simulink model "test_model"  (R2019b)
settings: Solver=VariableStepAuto  StartTime=0.0  StopTime=20  RelTol=1e-5
values from neighbouring files (symbols this model uses):
  dq0 = optimization(4:6)    [run_optimization.m]    (also in run_simulation.m = [0; 0; 8]; set_path.m = [0; 0; 8]; test_simulink.m = [0; 0; 8])
  q0 = optimization(1:3)    [run_optimization.m]    (also in run_simulation.m = [pi/9; -pi/9; 0]; set_path.m = [pi/9; -pi/9; 0]; test_simulink.m = [pi/9; -pi/9; 0])
  threshold = 1e-3    (= 0.001)    [test_simulink.m]
  x0 = [q0;dq0]    [set_path.m]    (also in test_simulink.m)
libraries: dspinverses x1
settings Model: Creator=Niilouf  LastModifiedBy=berth

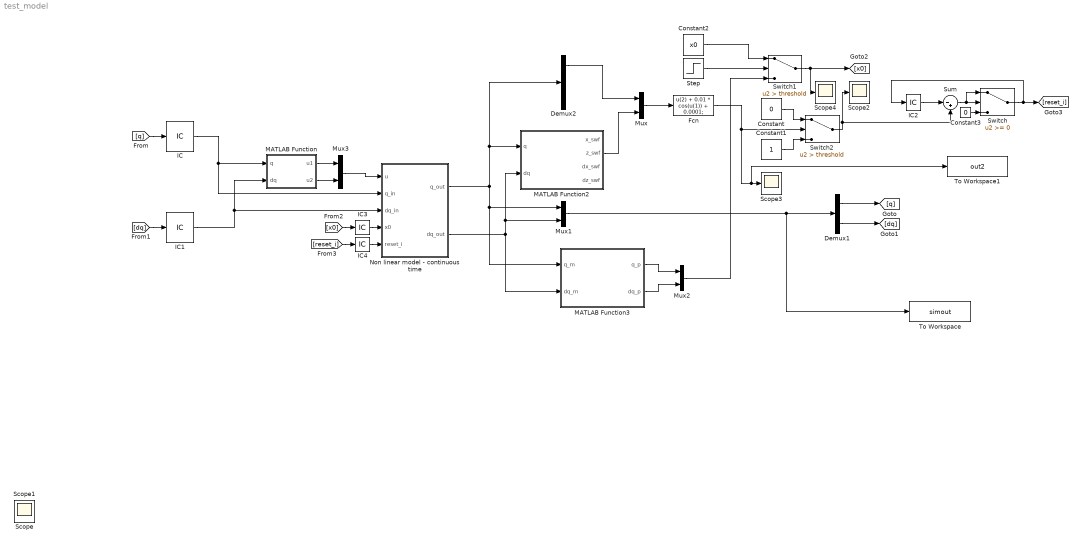
== system test_model ==
  Constant : Constant  Value=0
  Constant1 : Constant
  Constant2 : Constant  Value=x0
  Constant3 : Constant  Value=0
  Demux1 : Demux  Outputs=2
  Demux2 : Demux  Outputs=3
  Fcn : Fcn  Expr=u(2) + 0.01 * cos(u(1)) + 0.0001;
  IC : InitialCondition  Value=q0
  IC1 : InitialCondition  Value=dq0
  IC2 : InitialCondition  Value=0
  IC3 : InitialCondition  Value=x0
  IC4 : InitialCondition  Value=0
  MATLAB Function : MATLAB Function  TreatAsAtomicUnit=on
  MATLAB Function2 : MATLAB Function  TreatAsAtomicUnit=on
  MATLAB Function3 : MATLAB Function  TreatAsAtomicUnit=on
  Mux{,1..3} (4 alike) : Mux  Inputs=2
  Non linear model - continuous time : Subsystem
  Scope{,1..4} (5 alike) : Scope
  Step : Step  Time=1e-5  Before=1  After=0  SampleTime=0
  Sum : Sum  Inputs=|-+
  Switch : Switch
  Switch1 : Switch  Criteria=u2 > Threshold  Threshold=threshold
  Switch2 : Switch  Criteria=u2 > Threshold  Threshold=threshold
  To Workspace : ToWorkspace  VariableName=simout  SaveFormat=Timeseries  SampleTime=-1
  To Workspace1 : ToWorkspace  VariableName=out2  SaveFormat=Structure With Time  SampleTime=-1
  wires:
  Non linear model - continuous time/2(dq_out) -> Mux1/2, MATLAB Function2/2(dq), MATLAB Function3/2(dq_m)
  Non linear model - continuous time/1(q_out) -> MATLAB Function3/1(q_m), Mux1/1, MATLAB Function2/1(q), Demux2/1
  MATLAB Function2/2(z_swf) -> Mux/2
  Mux/1 -> Fcn/1
  Fcn/1 -> To Workspace1/1, Scope3/1, Switch2/2
  MATLAB Function3/1(q_p) -> Mux2/1
  MATLAB Function3/2(dq_p) -> Mux2/2
  Mux2/1 -> Switch1/3
  Mux1/1 -> To Workspace/1, Demux1/1
  Demux1/1 -> [q]
  Demux1/2 -> [dq]
  [q] -> IC/1
  [dq] -> IC1/1
  IC/1 -> MATLAB Function/1(q), Non linear model - continuous time/2(q_in)
  IC1/1 -> MATLAB Function/2(dq), Non linear model - continuous time/3(dq_in)
  MATLAB Function/1(u1) -> Mux3/1
  MATLAB Function/2(u2) -> Mux3/2
  Mux3/1 -> Non linear model - continuous time/1(u)
  Switch1/1 -> [x0], Scope4/1
  [x0] -> IC3/1
  Constant/1 -> Switch2/1
  Constant1/1 -> Switch2/3
  Switch2/1 -> Scope2/1, Sum/2
  [reset_i] -> IC4/1
  Demux2/1 -> Mux/1
  Constant2/1 -> Switch1/1
  Step/1 -> Switch1/2
  IC2/1 -> Sum/1
  Sum/1 -> Switch/1, Switch/2
  Constant3/1 -> Switch/3
  Switch/1 -> IC2/1, [reset_i]
  IC3/1 -> Non linear model - continuous time/4(x0)
  IC4/1 -> Non linear model - continuous time/5("reset_i ")

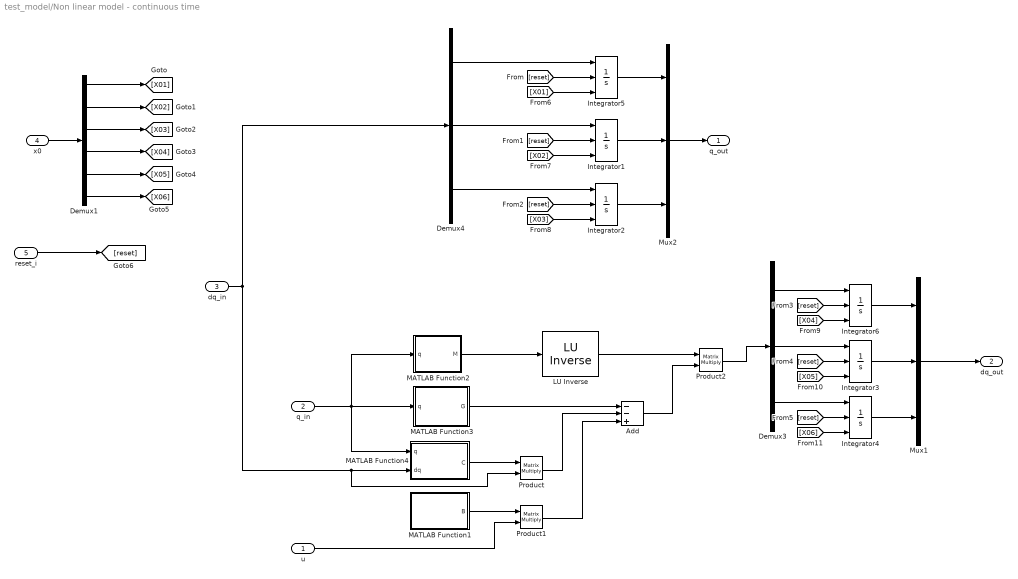
== system test_model/Non linear model - continuous time ==
  u : Inport  PortDimensions=2
  q_in : Inport  Port=2  PortDimensions=3
  dq_in : Inport  Port=3  PortDimensions=3
  x0 : Inport  Port=4  PortDimensions=6
  "reset_i " : Inport  Port=5
  " LU Inverse" : dspinverses/ LU Inverse
      settings: SourceProductName=DSP System Toolbox
  Add : Sum  Inputs=--+
  Demux1 : Demux  Outputs=6
  Demux3 : Demux  Outputs=3
  Demux4 : Demux  Outputs=3
  Integrator{1..6} (6 alike) : Integrator  ExternalReset=rising  InitialConditionSource=external  InitialCondition=x0(1)
  MATLAB Function1 : MATLAB Function  TreatAsAtomicUnit=on
  MATLAB Function2 : MATLAB Function  TreatAsAtomicUnit=on
  MATLAB Function3 : MATLAB Function  TreatAsAtomicUnit=on
  MATLAB Function4 : MATLAB Function  TreatAsAtomicUnit=on
  Mux1 : Mux  Inputs=3
  Mux2 : Mux  Inputs=3
  Product : Product  Multiplication=Matrix(*)
  Product1 : Product  Multiplication=Matrix(*)
  Product2 : Product  Multiplication=Matrix(*)
  q_out : Outport  PortDimensions=3  VectorParamsAs1DForOutWhenUnconnected=off
  dq_out : Outport  Port=2  PortDimensions=3  VectorParamsAs1DForOutWhenUnconnected=off
  wires:
  Demux4/1 -> Integrator5/1
  q_in/1 -> MATLAB Function2/1(q), MATLAB Function4/1(q), MATLAB Function3/1(q)
  Mux2/1 -> q_out/1
  dq_in/1 -> Demux4/1, MATLAB Function4/2(dq), Product/2
  Mux1/1 -> dq_out/1
  MATLAB Function4/1(C) -> Product/1
  MATLAB Function1/1(B) -> Product1/1
  MATLAB Function3/1(G) -> Add/1
  Product1/1 -> Add/3
  Product/1 -> Add/2
  Add/1 -> Product2/2
  Product2/1 -> Demux3/1
  MATLAB Function2/1(M) -> " LU Inverse"/1
  " LU Inverse"/1 -> Product2/1
  u/1 -> Product1/2
  Demux4/2 -> Integrator1/1
  Demux4/3 -> Integrator2/1
  x0/1 -> Demux1/1
  Demux3/1 -> Integrator6/1
  Integrator6/1 -> Mux1/1
  Integrator3/1 -> Mux1/2
  Integrator4/1 -> Mux1/3
  Demux3/2 -> Integrator3/1
  Demux3/3 -> Integrator4/1
  Integrator5/1 -> Mux2/1
  Integrator1/1 -> Mux2/2
  Integrator2/1 -> Mux2/3
  Demux1/1 -> [X01]
  Demux1/2 -> [X02]
  Demux1/3 -> [X03]
  Demux1/4 -> [X04]
  Demux1/5 -> [X05]
  Demux1/6 -> [X06]
  "reset_i "/1 -> [reset]
  [reset] -> Integrator5/2
  [reset] -> Integrator2/2
  [reset] -> Integrator1/2
  [X01] -> Integrator5/3
  [X03] -> Integrator2/3
  [X02] -> Integrator1/3
  [reset] -> Integrator6/2
  [X04] -> Integrator6/3
  [reset] -> Integrator3/2
  [reset] -> Integrator4/2
  [X05] -> Integrator3/3
  [X06] -> Integrator4/3

== matlab function test_model/MATLAB Function2 ==
  data: x_swf output; q input; dq input; z_swf output; dx_swf output; dz_swf output
function [x_swf, z_swf, dx_swf, dz_swf] = kin_swf(q, dq)

if nargin == 1
    dq = zeros(3, 1);
end

q1 = q(1);
dq1 = dq(1);
q2 = q(2);
dq2 = dq(2);

[~, ~, ~, l1, l2, ~, ~] = set_parameters();

x_swf = l1*sin(q1) - l2*sin(q2);
z_swf = l1*cos(q1) - l2*cos(q2);
dx_swf = dq1*l1*cos(q1) - dq2*l2*cos(q2);
dz_swf = dq2*l2*sin(q2) - dq1*l1*sin(q1);

end

== matlab function test_model/MATLAB Function3 ==
  data: q_p output; q_m input; dq_m input; dq_p output
function [q_p, dq_p] = impact(q_m, dq_m)

q_p = zeros(3,1);

q_p(1, 1) = q_m(2);
q_p(2, 1) = q_m(1);
q_p(3, 1) = q_m(3);

A_m = eval_A_m(q_m);
A_p = eval_A_p(q_p);

% A_p dq_p = A_m dq_m
dq_p = A_p \ (A_m * dq_m);

end

== matlab function test_model/MATLAB Function ==
  data: u1 output; u2 output; q input; dq input
function [u1, u2]= control(q, dq)
% You may call control_hyper_parameters and desired_outputs in this function
% you don't necessarily need to use all the inputs to this control function

% extract parameters
kp1 = 457.5;
kp2 = 161;
kd1 = 77.05; 
kd2 = 5;
alpha = 10.4 * pi / 180;

% controller for torso
u1 = kp1*q(3)-alpha + kd1*dq(3);

% controller for legs
u2 = -kp2*(q(2)+q(1)) - kd2*(dq(2)+dq(1));

% saturate the output torque
u = [u1; u2];
u = max(min(u, 30), -30); 

u1 = u(1);
u2 = u(2);
end

== matlab function test_model/Non linear model - continuous time/MATLAB Function1 ==
  data: B output
function B = eval_B()
%EVAL_B
%    B = EVAL_B

%    This function was generated by the Symbolic Math Toolbox version 7.1.
%    14-Oct-2018 18:44:49

B = reshape([1.0,0.0,-1.0,0.0,1.0,-1.0],[3,2]);
end

== matlab function test_model/Non linear model - continuous time/MATLAB Function2 ==
  data: M output; q input
function M = eval_M(q)
%EVAL_M
%    M = EVAL_M(L1,L2,L3,M1,M2,M3,Q1,Q2,Q3)

%    This function was generated by the Symbolic Math Toolbox version 7.1.
%    14-Oct-2018 18:44:47
q1 = q(1);
q2 = q(2);
q3 = q(3);

[m1, m2, m3, l1, l2, l3, ~] = set_parameters();

t2 = q1-q2;
t3 = cos(t2);
t4 = q1-q3;
t5 = cos(t4);
t6 = l1.*l3.*m3.*t5.*(1.0./2.0);
M = reshape([l1.^2.*(m1.*(1.0./4.0)+m2+m3),l1.*l2.*m2.*t3.*(-1.0./2.0),t6,l1.*l2.*m2.*t3.*(-1.0./2.0),l2.^2.*m2.*(1.0./4.0),0.0,t6,0.0,l3.^2.*m3.*(1.0./4.0)],[3,3]);

== matlab function test_model/Non linear model - continuous time/MATLAB Function3 ==
  data: G output; q input
function G = eval_G(q)
%EVAL_G
%    G = EVAL_G(G,L1,L2,L3,M1,M2,M3,Q1,Q2,Q3)

%    This function was generated by the Symbolic Math Toolbox version 7.1.
%    14-Oct-2018 18:44:49
q1 = q(1);
q2 = q(2);
q3 = q(3);

[m1, m2, m3, l1, l2, l3, g] = set_parameters();

G = [g.*l1.*sin(q1).*(m1+m2.*2.0+m3.*2.0).*(-1.0./2.0);g.*l2.*m2.*sin(q2).*(1.0./2.0);g.*l3.*m3.*sin(q3).*(-1.0./2.0)];

== matlab function test_model/Non linear model - continuous time/MATLAB Function4 ==
  data: C output; q input; dq input
function C = eval_C(q, dq)
%EVAL_C
%    C = EVAL_C(DQ1,DQ2,DQ3,L1,L2,L3,M2,M3,Q1,Q2,Q3)

%    This function was generated by the Symbolic Math Toolbox version 7.1.
%    14-Oct-2018 18:44:48

q1 = q(1);
q2 = q(2);
q3 = q(3);
dq1 = dq(1);
dq2 = dq(2);
dq3 = dq(3);

[m1, m2, m3, l1, l2, l3, ~] = set_parameters();

t2 = q1-q2;
t3 = sin(t2);
t4 = q1-q3;
t5 = sin(t4);
C = reshape([0.0,dq1.*l1.*l2.*m2.*t3.*(1.0./2.0),dq1.*l1.*l3.*m3.*t5.*(-1.0./2.0),dq2.*l1.*l2.*m2.*t3.*(-1.0./2.0),0.0,0.0,dq3.*l1.*l3.*m3.*t5.*(1.0./2.0),0.0,0.0],[3,3]);
end
